simulink model "VehicleWithoutABS"  (R2014b)
settings: Solver=ode3  StartTime=0.0  StopTime=6  FixedStep=0.01  RelTol=1e-3
libraries: simulink x2
settings Model: Creator=树下曼荼罗  LastModifiedBy=树下曼荼罗

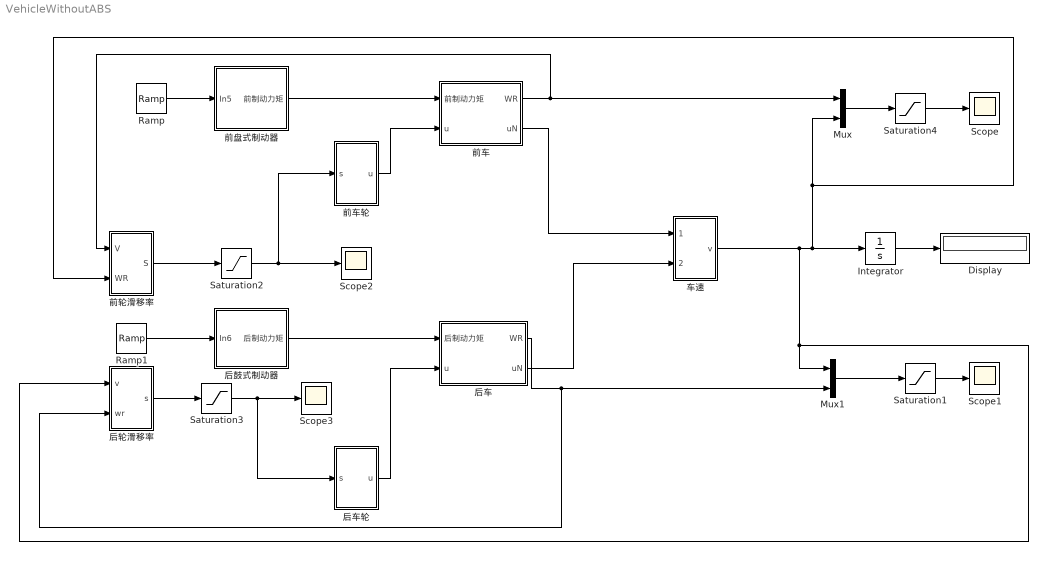
== system VehicleWithoutABS ==
  Display : Display
  Integrator : Integrator
  Mux : Mux  Inputs=2
  Mux1 : Mux  Inputs=2
  Ramp : simulink/Sources/Ramp  slope=1  start=0  X0=25
  Ramp1 : simulink/Sources/Ramp  slope=1  start=0  X0=10
  Saturation1 : Saturate  UpperLimit=25  LowerLimit=0
  Saturation2 : Saturate  UpperLimit=1  LowerLimit=0
  Saturation3 : Saturate  UpperLimit=1  LowerLimit=0
  Saturation4 : Saturate  UpperLimit=25  LowerLimit=0
  Scope{,1..3} (4 alike) : Scope
      Scope settings: ShowLegends=on  TimeRange=4  ScrollMode=on
      Scope1 settings: ShowLegends=on  TimeRange=4  YMin=-50  YMax=30  ScrollMode=on
      Scope2 settings: TimeRange=4  SaveName=ScopeData2
      Scope3 settings: TimeRange=4  SaveName=ScopeData3
  前盘式制动器 : Subsystem
  前车 : Subsystem
  前车轮 : Subsystem
  前轮滑移率 : Subsystem
  后车 : Subsystem
  后车轮 : Subsystem
  后轮滑移率 : Subsystem
  后鼓式制动器 : Subsystem
  车速 : Subsystem
  wires:
  后车轮/1(u) -> 后车/2(u)
  后车/1(WR) -> 后轮滑移率/2(wr), Mux1/2
  Integrator/1 -> Display/1
  Mux1/1 -> Saturation1/1
  Ramp/1 -> 前盘式制动器/1(In5)
  前盘式制动器/1(前制动力矩) -> 前车/1(前制动力矩)
  Ramp1/1 -> 后鼓式制动器/1(In6)
  后鼓式制动器/1(后制动力矩) -> 后车/1(后制动力矩)
  前车轮/1(u) -> 前车/2(u)
  前车/1(WR) -> 前轮滑移率/1(V), Mux/1
  Mux/1 -> Saturation4/1
  Saturation1/1 -> Scope1/1
  Saturation2/1 -> 前车轮/1(s), Scope2/1
  Saturation3/1 -> 后车轮/1(s), Scope3/1
  Saturation4/1 -> Scope/1
  车速/1(v) -> Mux1/1, 后轮滑移率/1(v), Mux/2, 前轮滑移率/2(WR), Integrator/1
  前车/2(uN) -> 车速/1(前uN)
  后车/2(uN) -> 车速/2(后uN)
  前轮滑移率/1(S) -> Saturation2/1
  后轮滑移率/1(s) -> Saturation3/1

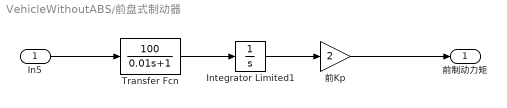
== system VehicleWithoutABS/前盘式制动器 ==
  In5 : Inport
  Integrator Limited1 : Integrator  UpperSaturationLimit=1  LowerSaturationLimit=0
  Transfer Fcn : TransferFcn  Numerator=[100]  Denominator=[0.01 1]
  前Kp : Gain  Gain=2
  前制动力矩 : Outport
  wires:
  前Kp/1 -> 前制动力矩/1
  In5/1 -> Transfer Fcn/1
  Transfer Fcn/1 -> Integrator Limited1/1
  Integrator Limited1/1 -> 前Kp/1

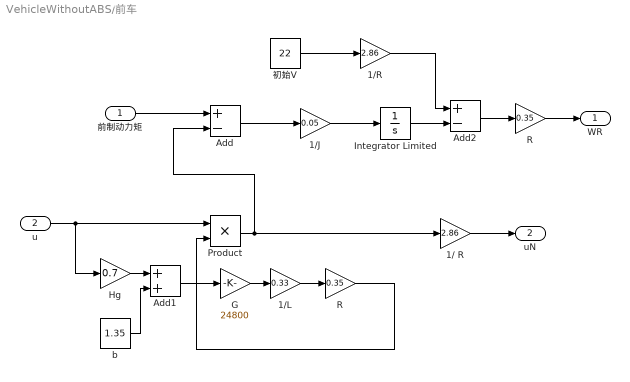
== system VehicleWithoutABS/前车 ==
  前制动力矩 : Inport
  u : Inport  Port=2
  1/ R : Gain  Gain=2.86
  1/J : Gain  Gain=0.05
  1/L : Gain  Gain=0.33
  1/R : Gain  Gain=2.86
  Add : Sum  Inputs=+-
  Add1 : Sum
  Add2 : Sum  Inputs=+-
  G : Gain  Gain=24800
  Hg : Gain  Gain=0.7
  Integrator Limited : Integrator  UpperSaturationLimit=1  LowerSaturationLimit=0
  Product : Product
  R : Gain  Gain=0.35
  "R " : Gain  Gain=0.35
  b : Constant  Value=1.35
  初始V : Constant  Value=22
  WR : Outport
  uN : Outport  Port=2
  wires:
  R/1 -> WR/1
  Add1/1 -> G/1
  Add/1 -> 1/J/1
  Product/1 -> Add/2, 1/ R/1
  b/1 -> Add1/2
  u/1 -> Hg/1, Product/1
  1/L/1 -> "R "/1
  G/1 -> 1/L/1
  Hg/1 -> Add1/1
  前制动力矩/1 -> Add/1
  "R "/1 -> Product/2
  1/J/1 -> Integrator Limited/1
  初始V/1 -> 1/R/1
  1/R/1 -> Add2/1
  Integrator Limited/1 -> Add2/2
  Add2/1 -> R/1
  1/ R/1 -> uN/1

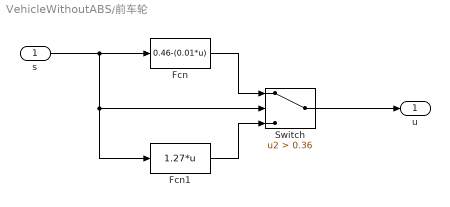
== system VehicleWithoutABS/前车轮 ==
  s : Inport
  Fcn : Fcn  Expr=0.46-(0.01*u)
  Fcn1 : Fcn  Expr=1.27*u
  Switch : Switch  Criteria=u2 > Threshold  Threshold=0.36
  u : Outport
  wires:
  s/1 -> Switch/2, Fcn1/1, Fcn/1
  Fcn/1 -> Switch/1
  Fcn1/1 -> Switch/3
  Switch/1 -> u/1

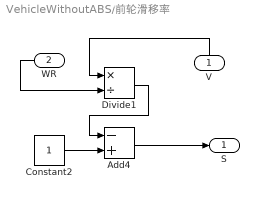
== system VehicleWithoutABS/前轮滑移率 ==
  V : Inport
  WR : Inport  Port=2
  Add4 : Sum  Inputs=-+
  Constant2 : Constant
  Divide1 : Product  Inputs=*/
  S : Outport
  wires:
  V/1 -> Divide1/1
  WR/1 -> Divide1/2
  Constant2/1 -> Add4/2
  Divide1/1 -> Add4/1
  Add4/1 -> S/1

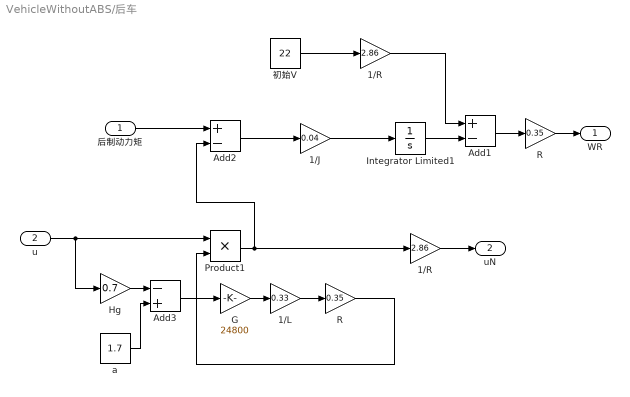
== system VehicleWithoutABS/后车 ==
  后制动力矩 : Inport
  u : Inport  Port=2
  1/J : Gain  Gain=0.04
  1/L : Gain  Gain=0.33
  1/R : Gain  Gain=2.86
  "1/R " : Gain  Gain=2.86
  Add1 : Sum  Inputs=+-
  Add2 : Sum  Inputs=+-
  Add3 : Sum  Inputs=-+
  G : Gain  Gain=24800
  Hg : Gain  Gain=0.7
  Integrator Limited1 : Integrator  UpperSaturationLimit=1  LowerSaturationLimit=0
  Product1 : Product
  R : Gain  Gain=0.35
  "R " : Gain  Gain=0.35
  a : Constant  Value=1.7
  初始V : Constant  Value=22
  WR : Outport
  uN : Outport  Port=2
  wires:
  Product1/1 -> "1/R "/1, Add2/2
  后制动力矩/1 -> Add2/1
  R/1 -> WR/1
  G/1 -> 1/L/1
  Add2/1 -> 1/J/1
  1/J/1 -> Integrator Limited1/1
  u/1 -> Hg/1, Product1/1
  Hg/1 -> Add3/1
  Add3/1 -> G/1
  1/L/1 -> "R "/1
  a/1 -> Add3/2
  "R "/1 -> Product1/2
  初始V/1 -> 1/R/1
  1/R/1 -> Add1/1
  Integrator Limited1/1 -> Add1/2
  Add1/1 -> R/1
  "1/R "/1 -> uN/1

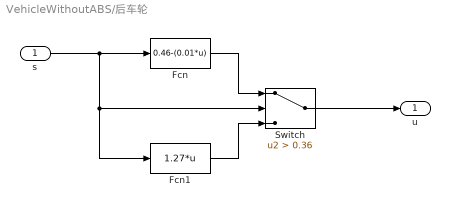
== system VehicleWithoutABS/后车轮 ==
  s : Inport
  Fcn : Fcn  Expr=0.46-(0.01*u)
  Fcn1 : Fcn  Expr=1.27*u
  Switch : Switch  Criteria=u2 > Threshold  Threshold=0.36
  u : Outport
  wires:
  s/1 -> Switch/2, Fcn1/1, Fcn/1
  Fcn/1 -> Switch/1
  Fcn1/1 -> Switch/3
  Switch/1 -> u/1

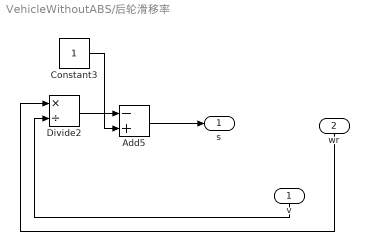
== system VehicleWithoutABS/后轮滑移率 ==
  v : Inport
  wr : Inport  Port=2
  Add5 : Sum  Inputs=-+
  Constant3 : Constant
  Divide2 : Product  Inputs=*/
  s : Outport
  wires:
  v/1 -> Divide2/2
  wr/1 -> Divide2/1
  Divide2/1 -> Add5/1
  Add5/1 -> s/1
  Constant3/1 -> Add5/2

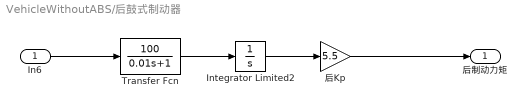
== system VehicleWithoutABS/后鼓式制动器 ==
  In6 : Inport
  Integrator Limited2 : Integrator  UpperSaturationLimit=1  LowerSaturationLimit=0
  Transfer Fcn : TransferFcn  Numerator=[100]  Denominator=[0.01 1]
  后Kp : Gain  Gain=5.5
  后制动力矩 : Outport
  wires:
  后Kp/1 -> 后制动力矩/1
  Transfer Fcn/1 -> Integrator Limited2/1
  Integrator Limited2/1 -> 后Kp/1
  In6/1 -> Transfer Fcn/1

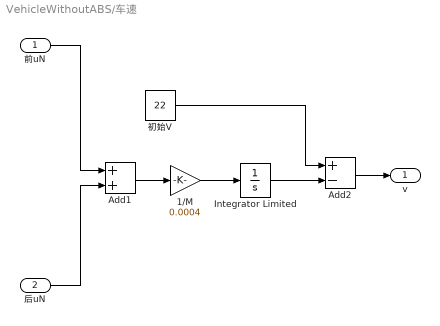
== system VehicleWithoutABS/车速 ==
  前uN : Inport
  后uN : Inport  Port=2
  1/M : Gain  Gain=0.0004
  Add1 : Sum
  Add2 : Sum  Inputs=+-
  Integrator Limited : Integrator  UpperSaturationLimit=1  LowerSaturationLimit=0
  初始V : Constant  Value=22
  v : Outport
  wires:
  Add2/1 -> v/1
  后uN/1 -> Add1/2
  Add1/1 -> 1/M/1
  Integrator Limited/1 -> Add2/2
  初始V/1 -> Add2/1
  1/M/1 -> Integrator Limited/1
  前uN/1 -> Add1/1
